simulink model "PrimaryStateMachine"  (R2024a)
settings: Solver=FixedStepDiscrete  StartTime=0.0  StopTime=20  FixedStep=.005  RelTol=1e-3
values from neighbouring files (symbols this model uses):
  StateReq : value not decoded    [Dictionary.sldd]
libraries: simulink x3
settings Model: DataDictionary=Dictionary.sldd  Creator=aloehr  LastModifiedBy=aloehr
settings SolverCC: AlgebraicLoopSolver=TrustRegion  PositivePriorityOrder=on
settings OptimizationCC: DefaultParameterBehavior=Inlined  UseDivisionForNetSlopeComputation=on  GainParamInheritBuiltInType=on  UseFloatMulNetSlope=on  DefaultUnderspecifiedDataType=single  InlineInvariantSignals=on  PassReuseOutputArgsAs=Individual arguments  ZeroExternalMemoryAtStartup=off  ZeroInternalMemoryAtStartup=off  NoFixptDivByZeroProtection=on  EfficientFloat2IntCast=on  LifeSpan=1  OptimizeBlockOrder=speed  DifferentSizesBufferReuse=on  EfficientTunableParamExpr=on
settings DebuggingCC: ParameterTunabilityLossMsg=error  UnconnectedInputMsg=warning  UnconnectedOutputMsg=warning  UnconnectedLineMsg=warning  SFUnexpectedBacktrackingDiag=warning  SFNoUnconditionalDefaultTransitionDiag=warning
settings HardwareCC: ProdBitPerPointer=32  ProdBitPerSizeT=32  ProdBitPerPtrDiffT=32  ProdLargestAtomicInteger=Long  ProdLargestAtomicFloat=Double  ProdWordSize=32  ProdLongLongMode=on  ProdHWDeviceType=ARM Compatible->ARM Cortex-M  TargetBitPerPointer=64  TargetBitPerSizeT=64  TargetBitPerPtrDiffT=64  TargetLongLongMode=on  TargetIntDivRoundTo=Zero  TargetEndianess=LittleEndian  TargetWordSize=64  TargetHWDeviceType=MATLAB Host  ProdEqTarget=off
settings ModelReferenceCC: EnableRefExpFcnMdlSchedulingChecks=on
settings SFSimCC: MATLABDynamicMemAlloc=off
settings RTWCC: Description=Embedded Coder  SystemTargetFile=ert.tlc  GenCodeOnly=on  TemplateMakefile=ert_default_tmf  GenerateReport=on  Toolchain=GNU Tools for ARM Embedded Processors  BuildConfiguration=Debug  IncludeHyperlinkInReport=on  LaunchReport=on  DataTypeReplacement=CDataTypesFixedWidth  GenerateTraceInfo=on  GenerateTraceReport=on  GenerateTraceReportSl=on  GenerateTraceReportSf=on  GenerateTraceReportEml=on  GenerateCodeMetricsReport=on  GPUComputeCapability=3.5
settings CodeAppCC: ForceParamTrailComments=on  IgnoreCustomStorageClasses=off  OperatorAnnotations=on  SimulinkDataObjDesc=on  SFDataObjDesc=on  CustomSymbolStrGlobalVar=rt$N$M  CustomSymbolStrType=$N$M  CustomSymbolStrFcn=$N$M$F  CustomSymbolStrMacro=$N$M  InsertBlockDesc=on  EnableCustomComments=on  ReqsInCode=on
settings ERTTargetCC: TargetLangStandard=C99 (ISO)  GenerateSampleERTMain=on  IncludeMdlTerminateFcn=off  CombineSignalStateStructs=on  SupportAbsoluteTime=off  CodeInterfacePackaging=Reusable function  SupportComplex=off  SupportNonInlinedSFcns=on  InlinedParameterPlacement=NonHierarchical  ERTCustomFileTemplate=example_file_process.tlc  MaxIdInt64=INT64_MAX  MinIdInt64=INT64_MIN  MaxIdUint64=UINT64_MAX  MaxIdInt32=INT32_MAX  MinIdInt32=INT32_MIN  MaxIdUint32=UINT32_MAX  MaxIdInt16=INT16_MAX  MinIdInt16=INT16_MIN  MaxIdUint16=UINT16_MAX  MaxIdInt8=INT8_MAX  MinIdInt8=INT8_MIN  MaxIdUint8=UINT8_MAX

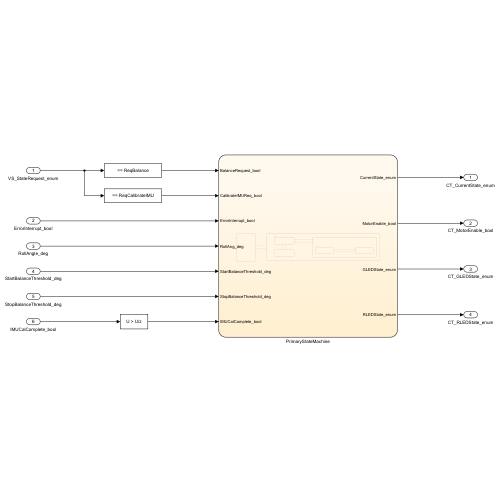
[thumbnail: Simulink's stored preview of the top-level diagram]
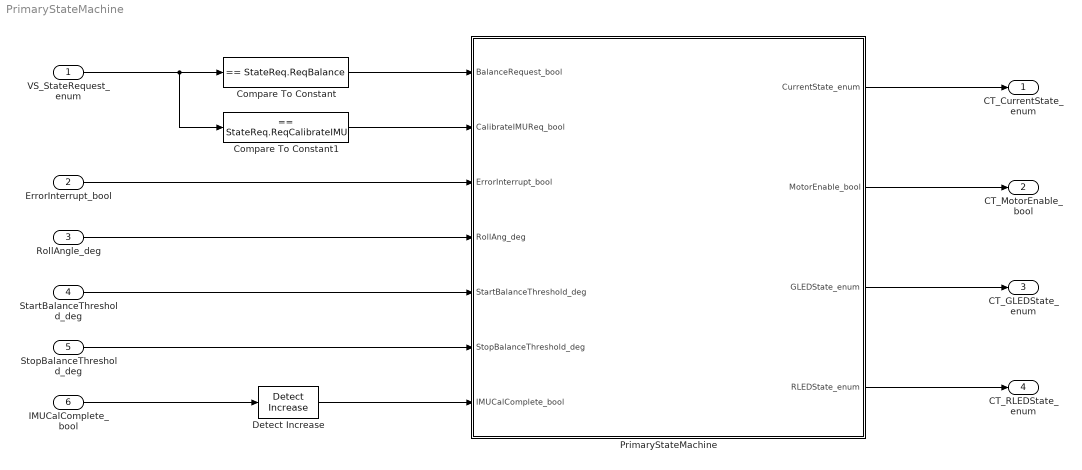
== system PrimaryStateMachine ==
  VS_StateRequest_enum : Inport  OutDataTypeStr=Enum: StateReq
  ErrorInterrupt_bool : Inport  Port=2  OutDataTypeStr=boolean
  RollAngle_deg : Inport  Port=3  OutDataTypeStr=single
  StartBalanceThreshold_deg : Inport  Port=4  OutDataTypeStr=single
  StopBalanceThreshold_deg : Inport  Port=5  OutDataTypeStr=single
  IMUCalComplete_bool : Inport  Port=6  OutDataTypeStr=boolean
  Compare To Constant : simulink/Logic and Bit Operations/Compare To Constant  relop===  const=StateReq.ReqBalance  OutDataTypeStr=boolean
  Compare To Constant1 : simulink/Logic and Bit Operations/Compare To Constant  relop===  const=StateReq.ReqCalibrateIMU  OutDataTypeStr=boolean
  Detect Increase : simulink/Logic and Bit Operations/Detect Increase  vinit=0.0  OutDataTypeStr=boolean
  PrimaryStateMachine : Stateflow chart  TreatAsAtomicUnit=on
  CT_CurrentState_enum : Outport  OutDataTypeStr=Enum: PrimaryState
  CT_MotorEnable_bool : Outport  Port=2  OutDataTypeStr=boolean
  CT_GLEDState_enum : Outport  Port=3  OutDataTypeStr=Enum: LEDState
  CT_RLEDState_enum : Outport  Port=4  OutDataTypeStr=Enum: LEDState
  wires:
  VS_StateRequest_enum/1 -> Compare To Constant/1, Compare To Constant1/1
  IMUCalComplete_bool/1 -> Detect Increase/1
  StopBalanceThreshold_deg/1 -> PrimaryStateMachine/6(StopBalanceThreshold_deg)
  Detect Increase/1 -> PrimaryStateMachine/7(IMUCalComplete_bool)
  Compare To Constant/1 -> PrimaryStateMachine/1(BalanceRequest_bool)
  ErrorInterrupt_bool/1 -> PrimaryStateMachine/3(ErrorInterrupt_bool)
  Compare To Constant1/1 -> PrimaryStateMachine/2(CalibrateIMUReq_bool)
  StartBalanceThreshold_deg/1 -> PrimaryStateMachine/5(StartBalanceThreshold_deg)
  RollAngle_deg/1 -> PrimaryStateMachine/4(RollAng_deg)
  PrimaryStateMachine/1(CurrentState_enum) -> CT_CurrentState_enum/1
  PrimaryStateMachine/4(RLEDState_enum) -> CT_RLEDState_enum/1
  PrimaryStateMachine/2(MotorEnable_bool) -> CT_MotorEnable_bool/1
  PrimaryStateMachine/3(GLEDState_enum) -> CT_GLEDState_enum/1

== stateflow chart PrimaryStateMachine/PrimaryStateMachine ==
  state Normal
    state Standby
      en:
      MotorEnable_bool = false;
      CurrentState_enum = PrimaryState.Standby;
      RLEDState_enum = LEDState.Off;
      GLEDState_enum = LEDState.On;
    state MotorEnabled
      en:
      MotorEnable_bool = true;
      RLEDState_enum = LEDState.Off;
      GLEDState_enum = LEDState.Blink;
      ex:
      MotorEnable_bool = false;
      state Balance
        en:
        CurrentState_enum = PrimaryState.Balance;
      state JumpUp
        en:
        CurrentState_enum = PrimaryState.JumpUp;
      (default) -> JumpUp
      JumpUp -> Balance : [abs(RollAng_deg) < StartBalanceThreshold_deg]
      Balance -> JumpUp : [abs(RollAng_deg) > StopBalanceThreshold_deg]
    state CalibrateIMU
      en:
      CurrentState_enum = PrimaryState.CalibrateIMU;
      RLEDState_enum = LEDState.Blink;
      GLEDState_enum = LEDState.Blink;
    (default) -> Standby
    Standby -> MotorEnabled [order 1] : [BalanceRequest_bool]
    MotorEnabled -> Standby : [~BalanceRequest_bool]
    Standby -> CalibrateIMU [order 2] : [CalibrateIMUReq_bool]
    CalibrateIMU -> Standby : [IMUCalComplete_bool]
  state Error
    en:
    MotorEnable_bool = false;
    CurrentState_enum = PrimaryState.Error;
    RLEDState_enum = LEDState.On;
    GLEDState_enum = LEDState.Off;
  (default) -> Normal
  Normal -> Error : [ErrorInterrupt_bool]
  Error -> Normal : [~ErrorInterrupt_bool]
  data: BalanceRequest_bool input boolean; CalibrateIMUReq_bool input boolean; ErrorInterrupt_bool input boolean; RollAng_deg input single; StartBalanceThreshold_deg input single; StopBalanceThreshold_deg input single; IMUCalComplete_bool input boolean; CurrentState_enum output Enum: PrimaryState =PrimaryState.Standby; MotorEnable_bool output boolean =false; GLEDState_enum output Enum: LEDState =LEDState.Off; RLEDState_enum output Enum: LEDState =LEDState.Off
